simulink model "onedof"  (R2021b)
settings: Solver=VariableStepAuto  StartTime=0.0  StopTime=10.0  RelTol=1e-3
settings Model: Creator=Emre  LastModifiedBy=Emre

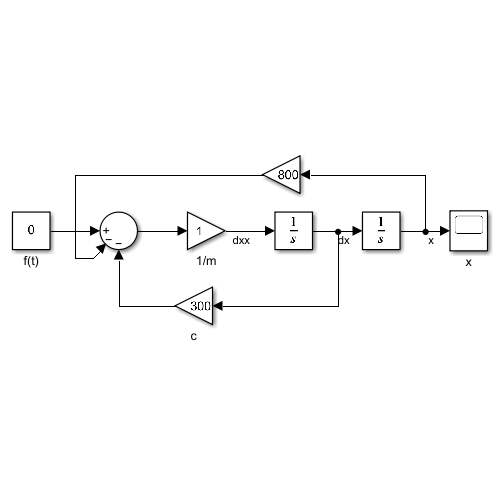
[thumbnail: Simulink's stored preview of the top-level diagram]
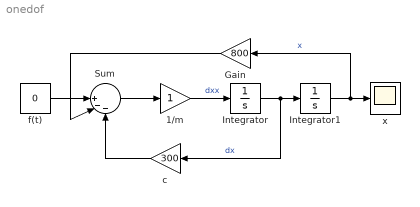
== system onedof ==
  1/m : Gain
  Gain : Gain  Gain=800
  Integrator : Integrator
  Integrator1 : Integrator
  Sum : Sum  Inputs=||+--
  c : Gain  Gain=300
  f(t) : Constant  Value=0
  x : Scope
  wires:
  Integrator1/1 -> x/1, Gain/1  "x"
  Gain/1 -> Sum/2
  Integrator/1 -> Integrator1/1, c/1  "dx"
  f(t)/1 -> Sum/1
  c/1 -> Sum/3
  1/m/1 -> Integrator/1  "dxx"
  Sum/1 -> 1/m/1
